simulink model "Reg_Int_Estim"  (R2021a)
settings: Solver=FixedStepAuto  StartTime=0.0  StopTime=tf  FixedStep=Ts  RelTol=1e-3
undefined symbols (not defined in the file): N, Noise, P, Q, Ts
libraries: simulink x1
settings Model: Creator=perruquetti  LastModifiedBy=perruquetti

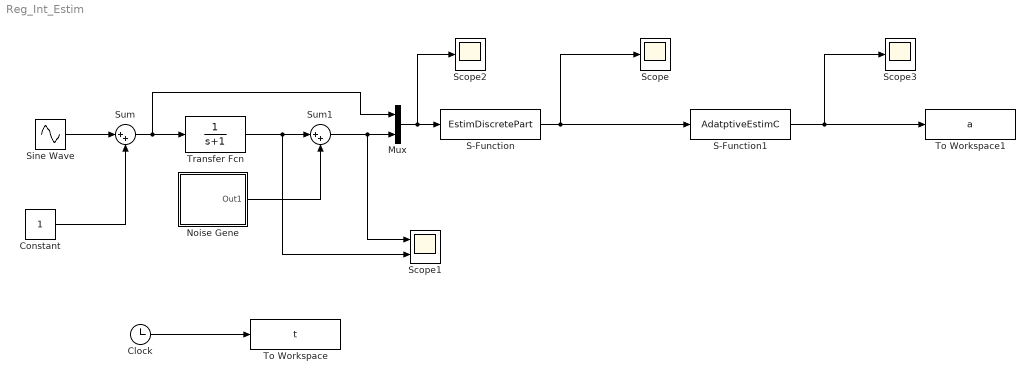
== system Reg_Int_Estim ==
  Clock : Clock
  Constant : Constant
  Mux : Mux  Inputs=2
  Noise Gene : Subsystem
  S-Function : S-Function  FunctionName=EstimDiscretePart  Parameters=N,Ts  SFunctionDeploymentMode=off  EnableBusSupport=off
  S-Function1 : S-Function  FunctionName=AdatptiveEstimC  Parameters=N,Ts,P,Q  SFunctionDeploymentMode=off  EnableBusSupport=off
  Scope : Scope
  Scope1 : Scope  NumInputPorts=2
  Scope2 : Scope
  Scope3 : Scope
  Sine Wave : Sin  Frequency=10  SampleTime=0
  Sum : Sum  Inputs=|++
  Sum1 : Sum  Inputs=|++
  To Workspace : ToWorkspace  VariableName=t  SampleTime=-1
  To Workspace1 : ToWorkspace  VariableName=a  SampleTime=-1
  Transfer Fcn : TransferFcn  Denominator=[1 1]  ParameterTunability=Unconstrained
  wires:
  Constant/1 -> Sum/2
  Sine Wave/1 -> Sum/1
  Sum/1 -> Transfer Fcn/1, Mux/1
  Clock/1 -> To Workspace/1
  Mux/1 -> Scope2/1, S-Function/1
  S-Function/1 -> S-Function1/1, Scope/1
  S-Function1/1 -> Scope3/1, To Workspace1/1
  Sum1/1 -> Scope1/1, Mux/2
  Transfer Fcn/1 -> Scope1/2, Sum1/1
  Noise Gene/1(Out1) -> Sum1/2

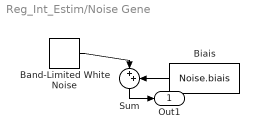
== system Reg_Int_Estim/Noise Gene ==
  Band-Limited White Noise : simulink/Sources/Band-Limited White Noise  Cov=Noise.power  Ts=Noise.sampling  seed=Noise.seed
  Biais : Constant  Value=Noise.biais
  Sum : Sum  Inputs=|++
  Out1 : Outport
  wires:
  Sum/1 -> Out1/1
  Biais/1 -> Sum/2
  Band-Limited White Noise/1 -> Sum/1
